simulink model "soc_wrapper_fpga"  (R2023b)
settings: Solver=FixedStepDiscrete  StartTime=0  StopTime=1000  FixedStep=1  RelTol=1e-3
settings Model: Creator=user poco smart  LastModifiedBy=user poco smart
settings SolverCC: AlgebraicLoopSolver=TrustRegion  PositivePriorityOrder=on  MinimalZcImpactIntegration=on
settings DataIOCC: SaveOutput=off  SaveTime=off  ReturnWorkspaceOutputs=off
settings OptimizationCC: DefaultParameterBehavior=Inlined  EnhancedBackFolding=on  PassReuseOutputArgsAs=Individual arguments  MaxStackSize=64  OptimizeBlockOrder=speed  DifferentSizesBufferReuse=on  OptimizationCustomize=off  EfficientTunableParamExpr=on
settings DebuggingCC: ParameterPrecisionLossMsg=none  ParameterTunabilityLossMsg=error  UnconnectedInputMsg=warning  UnconnectedOutputMsg=warning  UnconnectedLineMsg=warning  PregeneratedLibrarySubsystemCodeDiagnostic=none  ArithmeticOperatorsInVariantConditions=warning
settings HardwareCC: ProdBitPerPointer=32  ProdBitPerSizeT=32  ProdBitPerPtrDiffT=32  ProdLargestAtomicFloat=None  ProdIntDivRoundTo=Undefined  ProdEndianess=Unspecified  ProdWordSize=32  ProdHWDeviceType=ASIC/FPGA->ASIC/FPGA  TargetBitPerPointer=64  TargetBitPerSizeT=64  TargetBitPerPtrDiffT=64  TargetLongLongMode=on  TargetIntDivRoundTo=Zero  TargetEndianess=LittleEndian  TargetWordSize=64  TargetHWDeviceType=Custom Processor->MATLAB Host Computer  ProdEqTarget=off  HardwareBoardFeatureSet=SoCBlockset
settings ModelReferenceCC: EnableRefExpFcnMdlSchedulingChecks=on  ModelReferenceNumInstancesAllowed=Single
settings SFSimCC: SimUseLocalCustomCode=off  CustomCodeUndefinedFunction=UseInterfaceOnly
settings RTWCC: Description=Embedded Coder  SystemTargetFile=ert.tlc  HardwareBoard=Xilinx Zynq ZC706 evaluation kit  TLCOptions="-aInlineSetEventsForThisBaseRateFcn=TLC_FALSE -aSuppressMultiTaskScheduler=TLC_FALSE  -aRateBasedStepFcn=0"  TemplateMakefile=ert_default_tmf  GenerateReport=on  RTWUseLocalCustomCode=off  Toolchain=Linaro AArch32 Linux v6.3.1  IncludeHyperlinkInReport=on  LaunchReport=on  GenerateTraceInfo=on  GenerateTraceReport=on  GenerateTraceReportSl=on  GenerateTraceReportSf=on  GenerateTraceReportEml=on  DLArmComputeVersion=19.05
settings CodeAppCC: ForceParamTrailComments=on  IgnoreCustomStorageClasses=off  OperatorAnnotations=on  SimulinkDataObjDesc=on  SFDataObjDesc=on  InsertBlockDesc=on
settings ERTTargetCC: ExtModeTransport=2  ExtModeStaticAlloc=on  ExtModeMexFile=ext_xcp  ExtModeIntrfLevel=Level2 - Open
settings ConfigComp: CovBoundaryAbsTol=1.0e-5
settings SettingsController: UseSoCProfilerForTargets=0

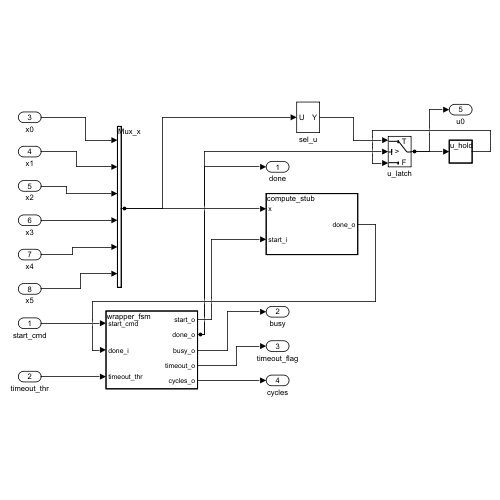
[thumbnail: Simulink's stored preview of the top-level diagram]
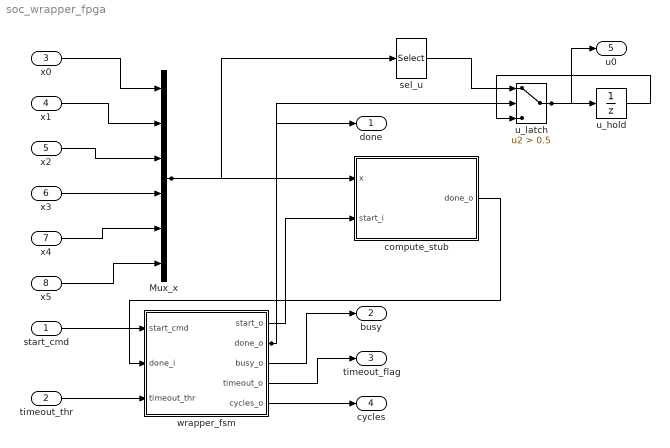
== system soc_wrapper_fpga ==
  start_cmd : Inport  OutDataTypeStr=boolean  PortDimensions=1
  timeout_thr : Inport  Port=2  OutDataTypeStr=uint32  PortDimensions=1
  x0 : Inport  Port=3  OutDataTypeStr=fixdt(1,32,16)  PortDimensions=1
  x1 : Inport  Port=4  OutDataTypeStr=fixdt(1,32,16)  PortDimensions=1
  x2 : Inport  Port=5  OutDataTypeStr=fixdt(1,32,16)  PortDimensions=1
  x3 : Inport  Port=6  OutDataTypeStr=fixdt(1,32,16)  PortDimensions=1
  x4 : Inport  Port=7  OutDataTypeStr=fixdt(1,32,16)  PortDimensions=1
  x5 : Inport  Port=8  OutDataTypeStr=fixdt(1,32,16)  PortDimensions=1
  Mux_x : Mux  Inputs=6
  compute_stub : MATLAB Function  TreatAsAtomicUnit=on
  sel_u : Selector  InputPortWidth=6  IndexOptions=Index vector (dialog)  Indices=1:1  OutputSizes=1
  u_hold : UnitDelay  SampleTime=-1
  u_latch : Switch  Criteria=u2 > Threshold  Threshold=0.5  SaturateOnIntegerOverflow=off  InputSameDT=off
  wrapper_fsm : MATLAB Function  TreatAsAtomicUnit=on
  done : Outport
  busy : Outport  Port=2
  timeout_flag : Outport  Port=3
  cycles : Outport  Port=4
  u0 : Outport  Port=5
  wires:
  u_latch/1 -> u_hold/1, u0/1
  x1/1 -> Mux_x/2
  x0/1 -> Mux_x/1
  u_hold/1 -> u_latch/3
  timeout_thr/1 -> wrapper_fsm/3(timeout_thr)
  x2/1 -> Mux_x/3
  x3/1 -> Mux_x/4
  x4/1 -> Mux_x/5
  x5/1 -> Mux_x/6
  start_cmd/1 -> wrapper_fsm/1(start_cmd)
  wrapper_fsm/2(done_o) -> u_latch/2, done/1
  Mux_x/1 -> compute_stub/1(x), sel_u/1
  wrapper_fsm/1(start_o) -> compute_stub/2(start_i)
  wrapper_fsm/3(busy_o) -> busy/1
  wrapper_fsm/4(timeout_o) -> timeout_flag/1
  wrapper_fsm/5(cycles_o) -> cycles/1
  sel_u/1 -> u_latch/1
  compute_stub/1(done_o) -> wrapper_fsm/2(done_i)

== matlab function soc_wrapper_fpga/compute_stub ==
  data: x input fixdt(1,32,16) size=6; done_o output boolean; start_i input boolean
function done_o = compute_stub(x, start_i) %#ok<INUSL>
%#codegen
% GENERATO DA build_wrapper_fpga.m — non modificare a mano.
%
% Segnaposto del blocco di calcolo di terzi. Latenza 500 cicli.
% NON e' un algoritmo: e' un ritardo con un handshake. Il calcolo
% vero e' di terzi e non e' nel nostro perimetro (docs/21_SPEC_WRAPPER §6).
%
% Il blocco e' configurato NONDIRECT FEEDTHROUGH: e' cio' che rompe
% l'anello fsm -> stub -> fsm senza aggiungere ritardi a mano.
% In cambio vale una regola, prescritta dalla documentazione HDL Coder:
%   "You must read the persistent variable's value BEFORE updating it."
% Le uscite si calcolano quindi in cima, dallo stato; gli aggiornamenti
% di stato stanno tutti dopo. Rompere questa regola non da' un errore:
% da' risultati sbagliati.
%
% Il segnaposto NON produce il dato: solo done. Il percorso dati va al
% latch del wrapper direttamente da x (docs/21_SPEC_WRAPPER §3). Serve
% perche' col nondirect feedthrough NESSUNA uscita puo' dipendere da un
% ingresso, e "u = x(1:nu)" ne dipenderebbe.
% x resta fra gli ingressi per fedelta' al contratto: il blocco vero lo
% legge, e deve poterlo fare in qualunque momento fra start e done.

    persistent cnt running doneReg
    LATENCY = uint32(500);
    if isempty(cnt)
        cnt     = uint32(0);
        running = false;
        doneReg = false;
    end

    % --- USCITE: solo dallo stato, prima di ogni aggiornamento ---
    done_o = doneReg;

    % --- AGGIORNAMENTI DI STATO ---
    doneReg = false;
    if running
        cnt = cnt + uint32(1);
        if cnt >= LATENCY
            running = false;
            doneReg = true;
        end
    elseif start_i
        running = true;
        cnt     = uint32(0);
    end
end

== matlab function soc_wrapper_fpga/wrapper_fsm ==
  data: start_cmd input boolean; start_o output boolean; done_i input boolean; timeout_thr input uint32; done_o output boolean; busy_o output boolean; timeout_o output boolean; cycles_o output uint32
function [start_o, done_o, busy_o, timeout_o, cycles_o] = wrapper_fsm(start_cmd, done_i, timeout_thr)
%#codegen
% GENERATO DA build_wrapper_fpga.m — non modificare a mano.

    persistent state cnt cyc doneL toL
    if isempty(state)
        state = uint8(0);   % 0=IDLE 1=RUNNING
        cnt   = uint32(0);
        cyc   = uint32(0);
        doneL = false;
        toL   = false;
    end

    start_o   = false;
    doneL     = false;   % DONE e TIMEOUT sono impulsi di un ciclo
    toL       = false;

    if state == uint8(0)
        % IDLE: si parte solo su comando. In RUNNING start_cmd e'
        % ignorato: un solve alla volta (I4).
        if start_cmd
            start_o = true;      % impulso di UN ciclo (I3)
            state   = uint8(1);
            cnt     = uint32(0);
        end
    else
        cnt = cnt + uint32(1);
        if done_i
            cyc   = cnt;         % latenza misurata (I5)
            doneL = true;
            state = uint8(0);
        elseif cnt >= timeout_thr
            cyc   = cnt;         % quanto si e' aspettato prima di mollare
            toL   = true;
            state = uint8(0);    % si esce SEMPRE (I6)
        end
    end

    done_o    = doneL;
    timeout_o = toL;
    busy_o    = (state == uint8(1));
    cycles_o  = cyc;
end
